simulink model "moj_statek"  (R2016a)
settings: Solver=VariableStepAuto  StartTime=0.0  StopTime=3000.0  RelTol=1e-3
settings Model: Creator=za32917  LastModifiedBy=za32917

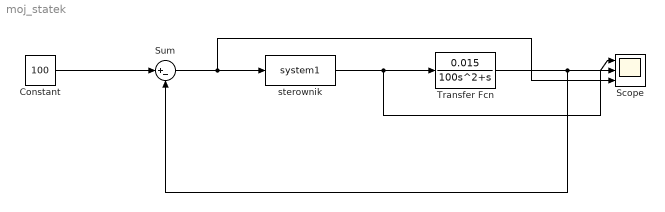
== system moj_statek ==
  Constant : Constant  Value=100
  Scope : Scope  NumInputPorts=3
  Sum : Sum  Inputs=|+-
  Transfer Fcn : TransferFcn  Numerator=0.015  Denominator=[100,1,0]
  "sterownik " : MATLABFcn  MATLABFcn=system1
  wires:
  "sterownik "/1 -> Scope/2, Transfer Fcn/1
  Transfer Fcn/1 -> Sum/2, Scope/1
  Constant/1 -> Sum/1
  Sum/1 -> Scope/3, "sterownik "/1
